simulink model "sampleModel46"  (R2021b)
settings: Solver=VariableStepAuto  StartTime=0.0  StopTime=10.0  RelTol=1e-3
undefined symbols (not defined in the file or in its folder): DiscIntNeverNeededParam
libraries: simulink x4
settings Model: Creator=user  LastModifiedBy=user

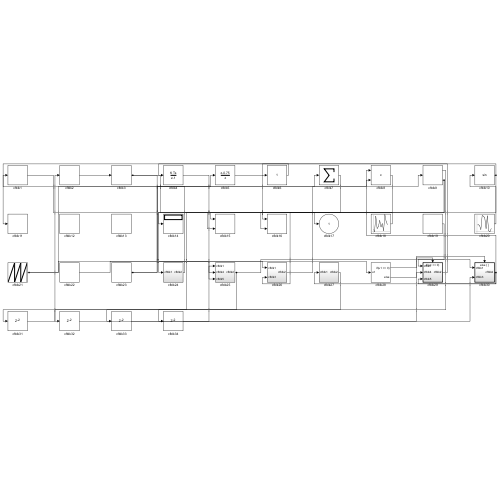
[thumbnail: Simulink's stored preview of the top-level diagram]
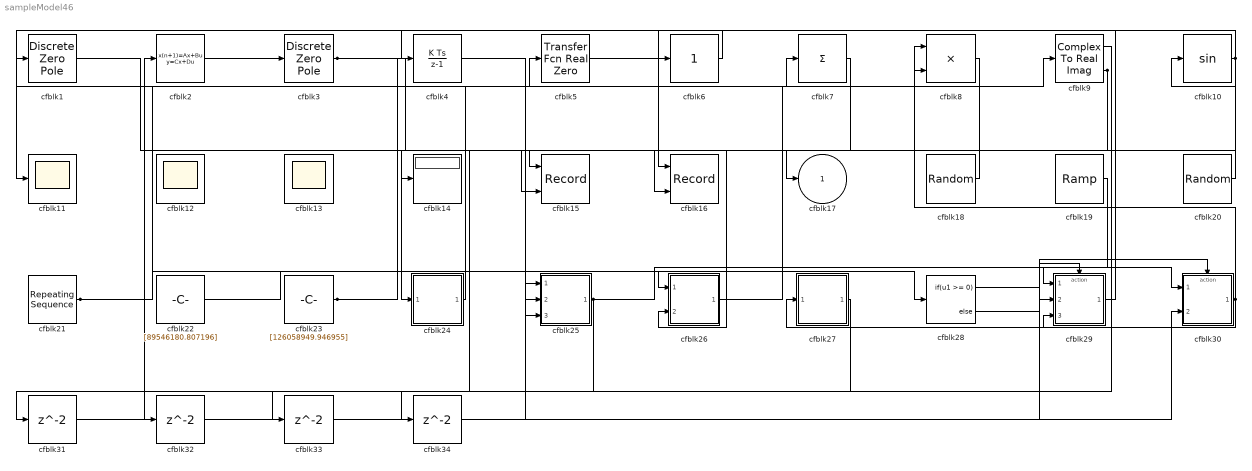
== system sampleModel46 ==
  cfblk1 : DiscreteZeroPole  Poles=[0 0.5]  Gain=1
  cfblk10 : Trigonometry
  cfblk11 : Scope
  cfblk12 : Scope
      settings: Floating=on
  cfblk13 : Scope
      settings: Floating=on
  cfblk14 : Display
  cfblk15 : Record  FileSettingsInternal="{\"entries\":[{\"content\":{\"excelSettings\":{\"content\":{},\"type\":\"Streamout.ExcelSettings\"}},\"type\":\"Streamout.FileSettingStorage\",\"uuid\":\"a4f2e3f9-dfc0-4756-a85c-d5ac2401a2c4\"}],\"packageUris\":[\"http://schema.mathworks.com/mf0/streamout_blocks/R2020a\"],\"version\":\"1.0\"}"  Layout=[1 1]  SignalsInternal="{\"entries\":[{\"content\":{\"signals\":[{\"content\":{\"blockPath\":[\"sampleModel46/cfblk15\"],\"channel\":[],\"dimensions\":[1],\"domain\":\"sampleModel46/cfblk15\",\"lineColor\":\"#a2142f\",\"plots\":[1],\"port\":1,\"sid\":[\"\"],\"signalID\":1777,\"signalName\":\"cfblk18\"},\"type\":\"RecordBlkView.Signal\",\"uuid\":\"71db0d78-ccd3-4ef5-aa7f-04574af591a6\"},{\"content\":{\"blockPath\":[\"sampleModel46/cfblk15\"],\"channel\":[],\"dimensions\":[1],\"domain\":\"sampleModel46/cfblk15\",\"lineColor\":\"#139fff\",\"plots\":[1],\"port\":2,\"sid\":[\"\"],\"signalID\":1781,\"signalName\":\"cfblk3\"},\"type\":\"RecordBlkView.Signal\",\"uuid\":\"4125a967-fd06-4072-b713-220b7ec39e00\"}]},\"type\":\"RecordBlkView.InputSignals\",\"uuid\":\"7bc6dbf7-48e5-4bde-9d9d-45c345172881\"}],\"packageUris\":[\"http://schema.mathworks.com/mf0/streamout_blocks/R2020a\"],\"version\":\"1.0\"}"  VisualizationBindings="{\"xyplotplugin\":{\"info\":[{\"series\":[{\"bindingParametersList\":[{\"parameter\":\"X-Axis\",\"signalID\":1777,\"signalName\":\"cfblk18\"},{\"parameter\":\"Y-Axis\",\"signalID\":1781,\"signalName\":\"cfblk3\"}],\"seriesID\":38232}],\"subplotID\":1}]}}"  CompatibilityTag=XY
  cfblk16 : Record  FileSettingsInternal="{\"entries\":[{\"content\":{\"excelSettings\":{\"content\":{},\"type\":\"Streamout.ExcelSettings\"}},\"type\":\"Streamout.FileSettingStorage\",\"uuid\":\"3210de24-3eb4-452b-a98a-413929911708\"}],\"packageUris\":[\"http://schema.mathworks.com/mf0/streamout_blocks/R2020a\"],\"version\":\"1.0\"}"  Layout=[1 1]  SignalsInternal="{\"entries\":[{\"content\":{\"signals\":[{\"content\":{\"blockPath\":[\"sampleModel46/cfblk16\"],\"channel\":[],\"dimensions\":[1],\"domain\":\"sampleModel46/cfblk16\",\"lineColor\":\"#a2142f\",\"plots\":[1],\"port\":1,\"sid\":[\"\"],\"signalID\":1785,\"signalName\":\"cfblk5\"},\"type\":\"RecordBlkView.Signal\",\"uuid\":\"2a312273-0dfb-470f-b63f-555e3245924f\"},{\"content\":{\"blockPath\":[\"sampleModel46/cfblk16\"],\"channel\":[],\"dimensions\":[1],\"domain\":\"sampleModel46/cfblk16\",\"lineColor\":\"#139fff\",\"plots\":[1],\"port\":2,\"sid\":[\"\"],\"signalID\":1789,\"signalName\":\"cfblk7\"},\"type\":\"RecordBlkView.Signal\",\"uuid\":\"6ec851d3-258b-4ded-9fb8-e1fe0cfdcc88\"}]},\"type\":\"RecordBlkView.InputSignals\",\"uuid\":\"893c7cfa-a348-4d41-9115-09620ed05e19\"}],\"packageUris\":[\"http://schema.mathworks.com/mf0/streamout_blocks/R2020a\"],\"version\":\"1.0\"}"  VisualizationBindings="{\"xyplotplugin\":{\"info\":[{\"series\":[{\"bindingParametersList\":[{\"parameter\":\"X-Axis\",\"signalID\":1785,\"signalName\":\"cfblk5\"},{\"parameter\":\"Y-Axis\",\"signalID\":1789,\"signalName\":\"cfblk7\"}],\"seriesID\":55971}],\"subplotID\":1}]}}"  CompatibilityTag=XY
  cfblk18 : UniformRandomNumber  Minimum=[-22822061.993170]  Maximum=[2682936175.554479]  Seed=[94614413.000000]  SampleTime=0.1
  cfblk19 : simulink/Sources/Ramp  slope=[-7757.447023]  start=[43.628253]  InitialOutput=[-780977.584783]
  cfblk2 : DiscreteStateSpace
  cfblk20 : RandomNumber  Mean=[79659.689950]  Variance=[63519.314613]  Seed=[600993799.000000]  SampleTime=0.1
  cfblk21 : simulink/Sources/Repeating Sequence  rep_seq_t=[0 2]  rep_seq_y=[-63156531.482019, 27809975.736590]
  cfblk22 : Constant  Value=[89546180.807196]  SampleTime=1
  cfblk23 : Constant  Value=[126058949.946955]  SampleTime=1
  cfblk24 : Subsystem
  cfblk25 : Subsystem
  cfblk26 : Subsystem
  cfblk27 : Subsystem
  cfblk28 : If  IfExpression=u1 >= 0  SampleTime=1
  cfblk29 : Subsystem  TreatAsAtomicUnit=on
  cfblk3 : DiscreteZeroPole  Poles=[0 0.5]  Gain=1
  cfblk30 : Subsystem  TreatAsAtomicUnit=on
  cfblk{31..34} (4 alike) : Delay  SampleTime=1
  cfblk4 : DiscreteIntegrator  ICPrevOutput=DiscIntNeverNeededParam  ICPrevScaledInput=DiscIntNeverNeededParam
  cfblk5 : simulink/Discrete/Transfer Fcn Real Zero  ZeroZ=0.75  ICPrevInput=0.0  DoSatur=off
      settings: SourceProductBaseCode=SL
  cfblk6 : simulink/Math Operations/Slider Gain  gain=1  low=0  high=2
  cfblk7 : Sum  Inputs=+
  cfblk8 : Product  Inputs=**
  cfblk9 : ComplexToRealImag
  cfblk17 : Outport
  wires:
  cfblk22/1 -> cfblk26/1(cfblk1)
  cfblk8/1 -> cfblk26/2(cfblk3)
  cfblk19/1 -> cfblk29/1(cfblk1)
  cfblk30/1(cfblk2) -> cfblk27/1(cfblk1), cfblk29/3(cfblk5), cfblk8/2
  cfblk18/1 -> cfblk15/1
  cfblk3/1 -> cfblk15/2, cfblk25/3(cfblk5)
  cfblk20/1 -> cfblk10/1
  cfblk21/1 -> cfblk28/1, cfblk8/1
  cfblk2/1 -> cfblk3/1
  cfblk5/1 -> cfblk16/1
  cfblk26/1(cfblk2) -> cfblk9/1
  cfblk7/1 -> cfblk16/2
  cfblk9/2 -> cfblk24/1(cfblk1), cfblk34/1
  cfblk25/1(cfblk2) -> cfblk30/1(cfblk1), cfblk31/1
  cfblk1/1 -> cfblk17/1
  cfblk4/1 -> cfblk25/2(cfblk4)
  cfblk29/1(cfblk2) -> cfblk11/1
  cfblk6/1 -> cfblk4/1
  cfblk24/1(cfblk2) -> cfblk1/1
  cfblk23/1 -> cfblk7/1, cfblk5/1
  cfblk10/1 -> cfblk14/1, cfblk6/1
  cfblk28/1 -> cfblk29/Action
  cfblk28/2 -> cfblk30/Action
  cfblk31/1 -> cfblk2/1
  cfblk27/1(cfblk2) -> cfblk32/1
  cfblk32/1 -> cfblk29/2(cfblk4)
  cfblk9/1 -> cfblk33/1
  cfblk33/1 -> cfblk25/1(cfblk1)
  cfblk34/1 -> cfblk30/2(cfblk3)

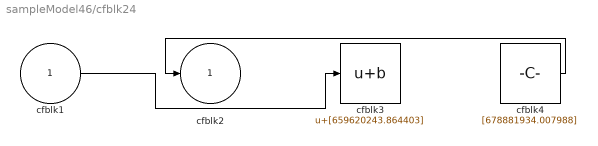
== system sampleModel46/cfblk24 ==
  cfblk1 : Inport
  cfblk3 : Bias  Bias=[659620243.864403]
  cfblk4 : Constant  Value=[678881934.007988]  SampleTime=1
  cfblk2 : Outport
  wires:
  cfblk4/1 -> cfblk2/1
  cfblk1/1 -> cfblk3/1

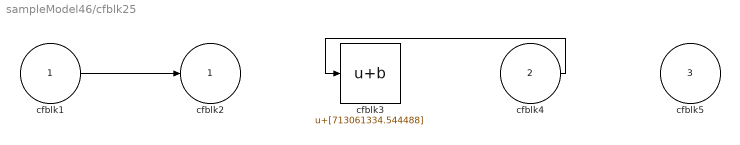
== system sampleModel46/cfblk25 ==
  cfblk1 : Inport
  cfblk4 : Inport  Port=2
  cfblk5 : Inport  Port=3
  cfblk3 : Bias  Bias=[713061334.544488]
  cfblk2 : Outport
  wires:
  cfblk4/1 -> cfblk3/1
  cfblk1/1 -> cfblk2/1

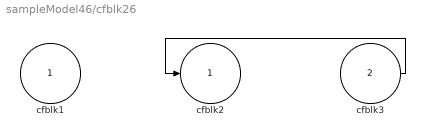
== system sampleModel46/cfblk26 ==
  cfblk1 : Inport
  cfblk3 : Inport  Port=2
  cfblk2 : Outport
  wires:
  cfblk3/1 -> cfblk2/1

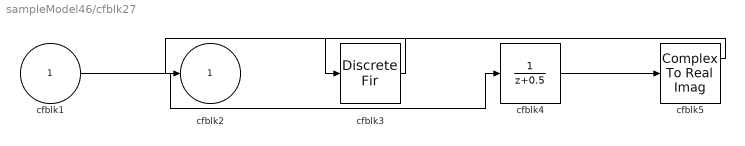
== system sampleModel46/cfblk27 ==
  cfblk1 : Inport
  cfblk3 : DiscreteFir  SampleTime=1
  cfblk4 : DiscreteTransferFcn  SampleTime=1
  cfblk5 : ComplexToRealImag
  cfblk2 : Outport
  wires:
  cfblk5/1 -> cfblk3/1
  cfblk4/1 -> cfblk5/1
  cfblk1/1 -> cfblk4/1
  cfblk3/1 -> cfblk2/1

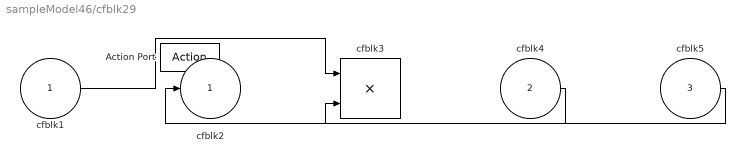
== system sampleModel46/cfblk29 ==
  cfblk1 : Inport
  cfblk4 : Inport  Port=2
  cfblk5 : Inport  Port=3
  Action Port : ActionPort  ActionPortLabel=if(u1 >= 0)
  cfblk3 : Product
  cfblk2 : Outport
  wires:
  cfblk5/1 -> cfblk2/1
  cfblk1/1 -> cfblk3/1
  cfblk4/1 -> cfblk3/2

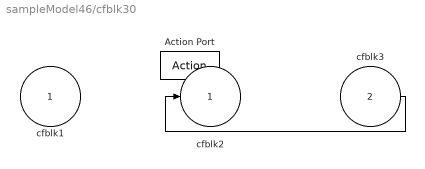
== system sampleModel46/cfblk30 ==
  cfblk1 : Inport
  cfblk3 : Inport  Port=2
  Action Port : ActionPort  ActionPortLabel=else
  cfblk2 : Outport
  wires:
  cfblk3/1 -> cfblk2/1
